simulink model "AC to AC converter"  (R2022b)
settings: Solver=VariableStepAuto  StartTime=0.0  StopTime=0.1  RelTol=1e-3
libraries: spsDiodeLib x8, spsThyristorLib x4, spsVoltageMeasurementLib x3, spsSeriesRLCBranchLib x2, spsACVoltageSourceLib x1, sps_lib x1
settings Model: Creator=alper  LastModifiedBy=alper

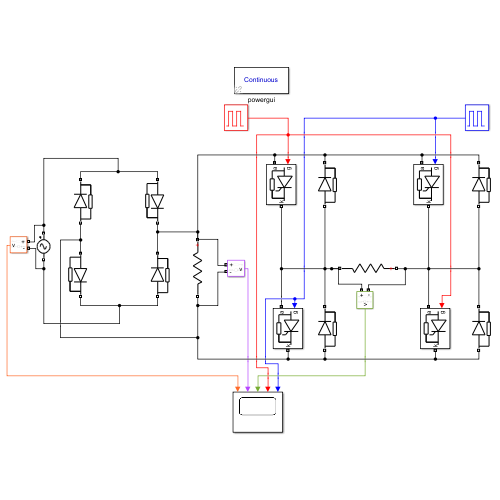
[thumbnail: Simulink's stored preview of the top-level diagram]
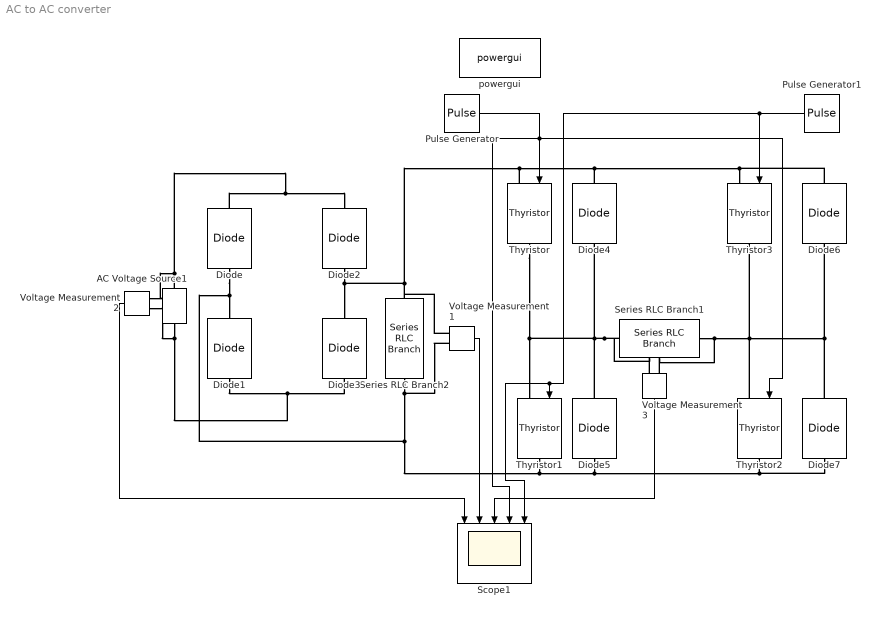
== system AC to AC converter ==
  AC Voltage Source1 : spsACVoltageSourceLib/AC Voltage Source  Amplitude=100  Phase=0  Frequency=50  SampleTime=0  Measurements=None  BusType=swing  Pref=10e3  Qref=0  Qmin=-inf  Qmax=+inf
  Diode{,1..7} (8 alike) : spsDiodeLib/Diode  Ron=0.001  Lon=0  Vf=0.8  IC=0  UseSnubber=0  Rs=500  Cs=250e-9  Measurements=off
  Pulse Generator : DiscretePulseGenerator  PulseType=Time based  Period=0.02  PulseWidth=50
  Pulse Generator1 : DiscretePulseGenerator  PulseType=Time based  Period=0.02  PulseWidth=50  PhaseDelay=0.01
  Scope1 : Scope  NumInputPorts=5
  Series RLC Branch1 : spsSeriesRLCBranchLib/Series RLC Branch  LConnTagsString=__new0  RConnTagsString=__new0  BranchType=R  Resistance=1  Inductance=1e-3  SetiL0=off  InitialCurrent=0  Capacitance=1e-6  Setx0=off  InitialVoltage=0  Measurements=None
  Series RLC Branch2 : spsSeriesRLCBranchLib/Series RLC Branch  LConnTagsString=__new0  RConnTagsString=__new0  BranchType=R  Resistance=1  Inductance=1e-3  SetiL0=off  InitialCurrent=0  Capacitance=1e-6  Setx0=off  InitialVoltage=0  Measurements=None
  Thyristor{,1..3} (4 alike) : spsThyristorLib/Thyristor  Ron=0.001  Lon=0  Vf=0.8  IC=0  Rs=500  Cs=250e-9  Measurements=off
  Voltage Measurement1 : spsVoltageMeasurementLib/Voltage Measurement  PhasorSimulation=off  OutputType=Complex  PSBequivalent=0
  Voltage Measurement2 : spsVoltageMeasurementLib/Voltage Measurement  PhasorSimulation=off  OutputType=Complex  PSBequivalent=0
  Voltage Measurement3 : spsVoltageMeasurementLib/Voltage Measurement  PhasorSimulation=off  OutputType=Complex  PSBequivalent=0
  powergui : sps_lib/powergui  Priority=1  SimulationMode=Continuous  SampleTime=50e-6  frequency=60  Iterations=50  frequencyindice=0  Pbase=100e6  ErrMax=1e-4  UnitsV=kV  UnitsW=MW  buscounter=0  FunctionMessages=off  echomessages=off  EnableUseOfTLC=off  CurrentSourceSwitches=off  DisableSnubberDevices=off  DisableRonSwitches=off  DisableVfSwitches=off  DisplayEquations=off  AutomaticDiscreteSolvers=off  SolverType=Tustin/Backward Euler (TBE)  Interpol=off  ExternalGateDelay=off  methode=off  Ts=100  x0status=blocks  SPID=on  SwTol=0  HookPort=off  NonlinearTolerance=1e-4  nMaxIteration=100  ContinueOnMaxIteration=off  RestoreLinks=warning  ResistiveCurrentMeasurement=off  Frange=[0:2:500]  Ylog=off  Xlog=on  ShowGrid=off  save=off  variable=ZData  structure=0  ZoomFFT=off  StartTime=0.0  cycles=1  DisplayStyle=1  fundamental=60  FreqAxis=off  MaxFrequency=1000  frequencyindicesteady=1  RmsSteady=1  display=off
  wires:
  Voltage Measurement3/1 -> Scope1/3
  Voltage Measurement1/1 -> Scope1/2
  Voltage Measurement2/1 -> Scope1/1
  Pulse Generator1/1 -> Scope1/5, Thyristor1/1, Thyristor3/1
  Pulse Generator/1 -> Thyristor2/1, Thyristor/1, Scope1/4
  connections:
  Thyristor/LConn1 -- Series RLC Branch2/LConn1 -- Voltage Measurement1/LConn1 -- Diode2/RConn1 -- Diode3/RConn1 -- Diode6/RConn1 -- Thyristor3/LConn1 -- Diode4/RConn1
  Series RLC Branch2/RConn1 -- Voltage Measurement1/LConn2 -- Diode/LConn1 -- Diode1/LConn1 -- Diode7/LConn1 -- Thyristor2/RConn1 -- Diode5/LConn1 -- Thyristor1/RConn1
  Diode7/RConn1 -- Diode6/LConn1 -- Thyristor2/LConn1 -- Voltage Measurement3/LConn2 -- Series RLC Branch1/LConn1 -- Thyristor3/RConn1
  Series RLC Branch1/RConn1 -- Diode5/RConn1 -- Diode4/LConn1 -- Thyristor1/LConn1 -- Thyristor/RConn1 -- Voltage Measurement3/LConn1
  AC Voltage Source1/LConn1 -- Diode1/RConn1 -- Diode3/LConn1 -- Voltage Measurement2/LConn2
  AC Voltage Source1/RConn1 -- Diode/RConn1 -- Diode2/LConn1 -- Voltage Measurement2/LConn1
